simulink model "TP_01_v18_01"  (R2018b)
settings: Solver=FixedStepAuto  StartTime=0.0  StopTime=15  FixedStep=0.01  RelTol=1e-3
settings Model: Creator=TMP  LastModifiedBy=TMP

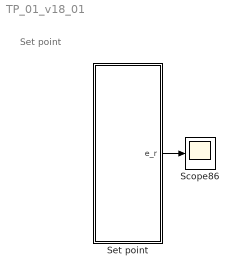
== system TP_01_v18_01 ==
  note: Set point
  Scope86 : Scope
  Set point : Subsystem
  wires:
  Set point/1(e_r) -> Scope86/1

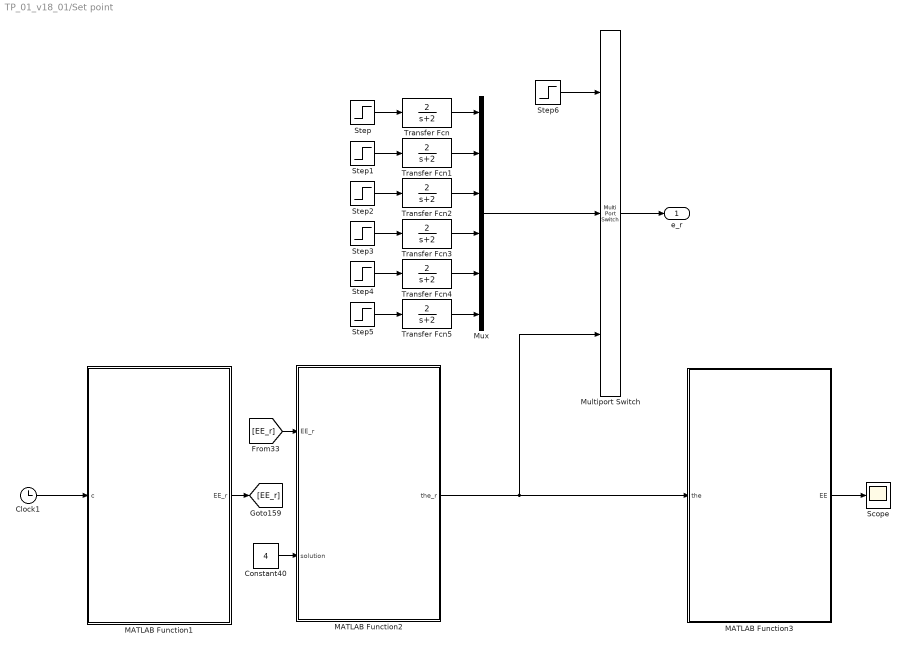
== system TP_01_v18_01/Set point ==
  Clock1 : Clock
  Constant40 : Constant  Value=4
  MATLAB Function1 : MATLAB Function  TreatAsAtomicUnit=on
  MATLAB Function2 : MATLAB Function  TreatAsAtomicUnit=on
  MATLAB Function3 : MATLAB Function  TreatAsAtomicUnit=on
  Multiport Switch : MultiPortSwitch  Inputs=2
  Mux : Mux  Inputs=6
  Scope : Scope
  Step : Step  Time=0  After=-0.052484081297928  SampleTime=0
  Step1 : Step  Time=0  After=0.010485739849624  SampleTime=0
  Step2 : Step  Time=0  After=0.105112260434987  SampleTime=0
  Step3 : Step  Time=0  After=-0.509342931142206  SampleTime=0
  Step4 : Step  Time=0  After=-0.649990510981055  SampleTime=0
  Step5 : Step  Time=0  After=-1.591522076129573  SampleTime=0
  Step6 : Step  Time=5  Before=1  After=2  SampleTime=0
  Transfer Fcn{,1..5} (6 alike) : TransferFcn  Numerator=[2]  Denominator=[1 2]
  e_r : Outport  VectorParamsAs1DForOutWhenUnconnected=off
  wires:
  Multiport Switch/1 -> e_r/1
  [EE_r] -> MATLAB Function2/1(EE_r)
  Clock1/1 -> MATLAB Function1/1(c)
  MATLAB Function1/1(EE_r) -> [EE_r]
  Constant40/1 -> MATLAB Function2/2(solution)
  Step/1 -> Transfer Fcn/1
  Step1/1 -> Transfer Fcn1/1
  Mux/1 -> Multiport Switch/2
  Step2/1 -> Transfer Fcn2/1
  Step3/1 -> Transfer Fcn3/1
  Step4/1 -> Transfer Fcn4/1
  Step5/1 -> Transfer Fcn5/1
  Transfer Fcn/1 -> Mux/1
  Transfer Fcn1/1 -> Mux/2
  Transfer Fcn2/1 -> Mux/3
  Transfer Fcn3/1 -> Mux/4
  Transfer Fcn4/1 -> Mux/5
  Transfer Fcn5/1 -> Mux/6
  Step6/1 -> Multiport Switch/1
  MATLAB Function2/1(the_r) -> MATLAB Function3/1(the), Multiport Switch/3
  MATLAB Function3/1(EE) -> Scope/1

== matlab function TP_01_v18_01/Set point/MATLAB Function1 ==
  data: c input; EE_r output
function EE_r = TrajectoryPlanning(c)
% H=ScopeData.signals.values(:,1:3);
t = c - 5;
f=0.1; %hz
Px_r = 450;
Py_r = 0+50*sin(2*pi*f*t);
Pz_r = 645+50*cos(2*pi*f*t);
roll_r=pi/3;
pitch_r=pi/6;
yaw_r=pi/2;
EE_r = [Px_r,Py_r,Pz_r,roll_r,pitch_r,yaw_r]';

== matlab function TP_01_v18_01/Set point/MATLAB Function2 ==
  data: EE_r input; the_r output; solution input
function the_r  = fcn(EE_r,solution)
a1=75; a2=270; a3=90; d1=335; d4=295; d7=80;
emt = zeros(8,6);
m = 0;
px = EE_r(1);
py = EE_r(2);
pz = EE_r(3);
roll = EE_r(4);
pitch = EE_r(5);
yaw =  EE_r(6);
r11 = cos(yaw)*cos(pitch);
r21 = sin(yaw)*cos(pitch);
r31 = -sin(pitch);
r12 = cos(yaw)*sin(pitch)*sin(roll) - sin(yaw)*cos(roll);
r22 = sin(yaw)*sin(pitch)*sin(roll) + cos(yaw)*cos(roll);
r32 = cos(pitch)*sin(roll);
r13 = cos(yaw)*sin(pitch)*cos(roll) + sin(yaw)*sin(roll);
r23 = sin(yaw)*sin(pitch)*cos(roll) - cos(yaw)*sin(roll);
r33 = cos(pitch)*cos(roll);
%% Inverse Kinematics
% Find the1
a_1 = py - r23*d7;
b_1 = - px + r13*d7;
d_1 = 0;
the11 = basic_01(a_1,b_1,d_1);

for i = 1:2
    % Find the2
    u = cos(the11(i))*(px-d7*r13) + sin(the11(i))*(py-r23*d7) - a1;
    v = pz - d1 - r33*d7;
    a_2 = v;
    b_2 = u;
    d_2 = (a3^2+d4^2-u^2-v^2-a2^2)/(-2*a2);
    the22 = basic_01(a_2,b_2,d_2);
    
    for j = 1:2
        % Find the3
        a_3 = a3;
        b_3 = d4;
        c_3 = u*sin(the22(j)) + v*cos(the22(j)) - a2;
        d_3 = u*cos(the22(j)) - v*sin(the22(j));
        the33 = basic_02(a_3,b_3,c_3,d_3);
        
        % Find the5
        c5 = (r13*cos(the11(i))*cos(the22(j)) - r33*sin(the22(j)) + r23*cos(the22(j))*sin(the11(i)))*cos(the33) - (r33*cos(the22(j)) + r13*cos(the11(i))*sin(the22(j)) + r23*sin(the11(i))*sin(the22(j)))*sin(the33);
        the55 = basic_01(1,0,c5);
        
        for k = 1:2
            % Find the4
            m = m+1;
            s4 = (r23*cos(the11(i)) - r13*sin(the11(i)))/(sin(the55(k)));
            c4 = (r33*cos(the22(j)) + r13*cos(the11(i))*sin(the22(j)) + r23*sin(the11(i))*sin(the22(j)) + sin(the33)*cos(the55(k))) / (-cos(the33)*sin(the55(k)));
            the44 = atan2(s4,c4);
            
            % Find the6
            a_6 = r21*cos(the11(i)) - r11*sin(the11(i));
            b_6 = r22*cos(the11(i)) - r12*sin(the11(i));
            c_6 = -sin(the44)*cos(the55(k));
            d_6 = cos(the44);
            the66 = basic_02(a_6,b_6,c_6,-d_6);
            emt(m,:)=[the11(i),the22(j),the33,the44,the55(k),the66];
        end
    end
end
% the = emt(solution,:);
the1 = emt(solution,1);
the2 = emt(solution,2);
the3 = emt(solution,3);
the4 = emt(solution,4);
the5 = emt(solution,5);
the6 = emt(solution,6);
the_r = [the1;the2;the3;the4;the5;the6];
end
function x = basic_01(a, b, d) % a*cos(x) + b*sin(x) = d
    anp = atan2(b, a);
    
    x1 = anp + atan2(sqrt(a*a + b*b - d*d), d);
    x2 = anp + atan2(-sqrt(a*a + b*b - d*d), d);
    x = [x1; x2];
end
function x = basic_02(a, b, c, d) 
    % a*cos(x) - b*sin(x) = c
    % b*cos(x) + a*sin(x) = d
    sinx = (d - b*c/a) / (b^2/a + a);
    cosx = (c + b*d/a) / (b^2/a + a);
    x = atan2(sinx,cosx);
end

== matlab function TP_01_v18_01/Set point/MATLAB Function3 ==
  data: the input; EE output
function EE  = FK_6DOF(the)
the1 = the(1);
the2 = the(2);
the3 = the(3);
the4 = the(4);
the5 = the(5);
the6 = the(6);
a1=75; a2=270; a3=90; d1=335; d4=295; d7=80;

T_0_EE = ...
[ cos(the6)*(cos(the5)*sin(the1)*sin(the4) + cos(the2 + the3)*cos(the1)*sin(the5) + cos(the1)*cos(the2)*cos(the4)*cos(the5)*sin(the3) + cos(the1)*cos(the3)*cos(the4)*cos(the5)*sin(the2)) - sin(the6)*(cos(the1)*cos(the2)*sin(the3)*sin(the4) - cos(the4)*sin(the1) + cos(the1)*cos(the3)*sin(the2)*sin(the4)), - cos(the6)*(cos(the1)*cos(the2)*sin(the3)*sin(the4) - cos(the4)*sin(the1) + cos(the1)*cos(the3)*sin(the2)*sin(the4)) - sin(the6)*(cos(the5)*sin(the1)*sin(the4) + cos(the2 + the3)*cos(the1)*sin(the5) + cos(the1)*cos(the2)*cos(the4)*cos(the5)*sin(the3) + cos(the1)*cos(the3)*cos(the4)*cos(the5)*sin(the2)), cos(the2 + the3)*cos(the1)*cos(the5) - sin(the5)*(sin(the1)*sin(the4) + cos(the1)*cos(the2)*cos(the4)*sin(the3) + cos(the1)*cos(the3)*cos(the4)*sin(the2)), a1*cos(the1) + a2*cos(the1)*sin(the2) + d4*cos(the1)*cos(the2)*cos(the3) + a3*cos(the1)*cos(the2)*sin(the3) + a3*cos(the1)*cos(the3)*sin(the2) - d4*cos(the1)*sin(the2)*sin(the3) - d7*sin(the1)*sin(the4)*sin(the5) + d7*cos(the1)*cos(the2)*cos(the3)*cos(the5) - d7*cos(the1)*cos(the5)*sin(the2)*sin(the3) - d7*cos(the1)*cos(the2)*cos(the4)*sin(the3)*sin(the5) - d7*cos(the1)*cos(the3)*cos(the4)*sin(the2)*sin(the5);
  cos(the6)*(cos(the2 + the3)*sin(the1)*sin(the5) - cos(the1)*cos(the5)*sin(the4) + cos(the2)*cos(the4)*cos(the5)*sin(the1)*sin(the3) + cos(the3)*cos(the4)*cos(the5)*sin(the1)*sin(the2)) - sin(the6)*(cos(the1)*cos(the4) + cos(the2)*sin(the1)*sin(the3)*sin(the4) + cos(the3)*sin(the1)*sin(the2)*sin(the4)), - cos(the6)*(cos(the1)*cos(the4) + cos(the2)*sin(the1)*sin(the3)*sin(the4) + cos(the3)*sin(the1)*sin(the2)*sin(the4)) - sin(the6)*(cos(the2 + the3)*sin(the1)*sin(the5) - cos(the1)*cos(the5)*sin(the4) + cos(the2)*cos(the4)*cos(the5)*sin(the1)*sin(the3) + cos(the3)*cos(the4)*cos(the5)*sin(the1)*sin(the2)), cos(the2 + the3)*cos(the5)*sin(the1) - sin(the5)*(cos(the2)*cos(the4)*sin(the1)*sin(the3) - cos(the1)*sin(the4) + cos(the3)*cos(the4)*sin(the1)*sin(the2)), a1*sin(the1) + a2*sin(the1)*sin(the2) + d4*cos(the2)*cos(the3)*sin(the1) + a3*cos(the2)*sin(the1)*sin(the3) + a3*cos(the3)*sin(the1)*sin(the2) + d7*cos(the1)*sin(the4)*sin(the5) - d4*sin(the1)*sin(the2)*sin(the3) + d7*cos(the2)*cos(the3)*cos(the5)*sin(the1) - d7*cos(the5)*sin(the1)*sin(the2)*sin(the3) - d7*cos(the2)*cos(the4)*sin(the1)*sin(the3)*sin(the5) - d7*cos(the3)*cos(the4)*sin(the1)*sin(the2)*sin(the5);
                                                                                                                                                                                          - cos(the6)*(sin(the2 + the3)*sin(the5) - cos(the2 + the3)*cos(the4)*cos(the5)) - cos(the2 + the3)*sin(the4)*sin(the6),                                                                                                                                                                                             sin(the6)*(sin(the2 + the3)*sin(the5) - cos(the2 + the3)*cos(the4)*cos(the5)) - cos(the2 + the3)*cos(the6)*sin(the4),                                                                                        - sin(the2 + the3)*cos(the5) - cos(the2 + the3)*cos(the4)*sin(the5),                                                                                                                                        d1 + a2*cos(the2) + a3*cos(the2)*cos(the3) - d4*cos(the2)*sin(the3) - d4*cos(the3)*sin(the2) - a3*sin(the2)*sin(the3) - d7*cos(the2)*cos(the5)*sin(the3) - d7*cos(the3)*cos(the5)*sin(the2) - d7*cos(the2)*cos(the3)*cos(the4)*sin(the5) + d7*cos(the4)*sin(the2)*sin(the3)*sin(the5);
                                                                                                                                                                                                                                                                                                               0,                                                                                                                                                                                                                                                                                                                0,                                                                                                                                                          0,                                                                                                                                                                                                                                                                                                                                                                                                                            1];
 
r11 = T_0_EE(1,1);
r21 = T_0_EE(2,1);
r31 = T_0_EE(3,1);
r12 = T_0_EE(1,2);
r22 = T_0_EE(2,2);
r32 = T_0_EE(3,2);
r13 = T_0_EE(1,3);
r23 = T_0_EE(2,3);
r33 = T_0_EE(3,3);
pitch = atan2(-r31,sqrt(r11^2+r21^2));
if pitch == pi/2
    yaw = 0;
    roll = atan2(r12,r22);
elseif pitch == -pi/2
    yaw = 0;
    roll = -atan2(r12,r22) ;     
else
    yaw = atan2(r21/cos(pitch),r11/cos(pitch));
    roll = atan2(r32/cos(pitch),r33/cos(pitch));
end
Px = T_0_EE(1,4);
Py = T_0_EE(2,4);
Pz = T_0_EE(3,4);
EE = [Px,Py,Pz,roll,pitch,yaw];
